simulink model "Vehicle_definitivo_validazione_2"  (R2025b)
settings: Solver=ode4  StartTime=0.0  StopTime=30  FixedStep=0.001  RelTol=1e-3
undefined symbols (not defined in the file): car, new_lotus_bump, new_lotus_roll, new_lotus_steer, posRef, rad, s, Tau_1, Tau_2, Tau_3, Tau_4, yawRef
libraries: aerolibconvert2 x28, simulink_extras x16, simulink x12, slpidlib x2, mpclib x1
(part 6 of 13)

== system Vehicle_definitivo_validazione_2/Con relaxation/Vehicle/Chassis/kinematics/FR ==
  note: mettere 2d su cmaber e toe
  Wheel_Travel : Inport
  Steer_Angle : Inport  Port=2
  Add : Sum
  Add1 : Sum  Inputs=+++
  Anti_dive : Lookup_n-D  NumberOfTableDimensions=1  BreakpointsForDimension1=[-20;-19;-18;-17;-16;-15;-14;-13;-12;-11;-10;-9;-8;-7;-6;-5;-4;-3;-2;-1;0;1;2;3;4;5;6;7;8;9;10;11;12;13;14;15;16;17;18;19;20;21;22;23;24;25;26;27;28;29;30;31;32;33;34;35;36;37;38;39;40;41;42;43;44;45;46;47;48;49;50;51;52;53;54;55;56;57;58;59;60;61;62;63;64;65;66;67;68;69;70;71;72;73;74;75]  Table=[53.85;54.03;54.22;54.4;54.59;54.77;54.96;55.15;55.34;55.53;55.72;55.92;56.11;56.31;56.5;56.7;56.9;57.1;57.3;57.5;57.71;57.91;58.12;58.32;58.53;58.74;58.95;59.16;59.38;59.59;59.81;60.03;60.24;60.46;60.69;60.91;61.13;61.36;61.59;61.81;62.04;62.28;62.51;62.74;62.98;63.22;63.46;63.7;63.94;64.18000000000001;64.43000000000001;64.68000000000001;64.92;65.17;65.43000000000001;65.68000000000001;65.94;66.19;66.45;66.72;66.98;67.23999999999999;67.51000000000001;67.78;68.05;68.31999999999999;68.59999999999999;68.87;69.15000000000001;69.43000000000001;69.72;70;70.29000000000001;70.58;70.87;71.16;71.45999999999999;71.75;72.05;72.36;72.66;72.97;73.28;73.59;73.91;74.22;74.54000000000001;74.86;75.19;75.52;75.84999999999999;76.18000000000001;76.51000000000001;76.84999999999999;77.19;77.54000000000001]/100  InternalRulePriority=Speed  RndMeth=Simplest
  Constant : Constant  Value=car.camber0_front
  Constant1 : Constant  Value=car.toe0_front
  Gain : Gain  Gain=0.222222
  IR : Lookup_n-D  NumberOfTableDimensions=1  BreakpointsForDimension1=[-20;-19;-18;-17;-16;-15;-14;-13;-12;-11;-10;-9;-8;-7;-6;-5;-4;-3;-2;-1;0;1;2;3;4;5;6;7;8;9;10;11;12;13;14;15;16;17;18;19;20;21;22;23;24;25;26;27;28;29;30;31;32;33;34;35;36;37;38;39;40;41;42;43;44;45;46;47;48;49;50;51;52;53;54;55;56;57;58;59;60;61;62;63;64;65;66;67;68;69;70;71;72;73;74;75]  Table=[0.556793;0.557414;0.558036;0.558659;0.559284;0.55991;0.5602240000000001;0.560538;0.561167;0.561167;0.561482;0.561798;0.562114;0.562114;0.562114;0.562114;0.562114;0.562114;0.562114;0.562114;0.561798;0.561798;0.561482;0.561482;0.561167;0.560852;0.560538;0.5602240000000001;0.55991;0.559284;0.558971;0.558347;0.558036;0.557414;0.557103;0.5564829999999999;0.555864;0.555247;0.554631;0.554017;0.553403;0.552792;0.552181;0.551572;0.550661;0.550055;0.549451;0.548546;0.547945;0.547046;0.546448;0.545554;0.544662;0.543774;0.543183;0.542299;0.541419;0.540541;0.539665;0.538793;0.537924;0.537057;0.536193;0.535332;0.534474;0.533618;0.532765;0.531915;0.531067;0.529942;0.529101;0.528262;0.527426;0.526593;0.525486;0.524659;0.523834;0.522739;0.521921;0.521105;0.5202909999999999;0.519211;0.5184029999999999;0.517598;0.516529;0.51573;0.514933;0.514139;0.513084;0.5122949999999999;0.511509;0.510725;0.509944;0.509165;0.508388;0.507614]  InternalRulePriority=Speed  RndMeth=Simplest
  camber : Lookup_n-D  NumberOfTableDimensions=1  BreakpointsForDimension1=[-20;-19;-18;-17;-16;-15;-14;-13;-12;-11;-10;-9;-8;-7;-6;-5;-4;-3;-2;-1;0;1;2;3;4;5;6;7;8;9;10;11;12;13;14;15;16;17;18;19;20;21;22;23;24;25;26;27;28;29;30;31;32;33;34;35;36;37;38;39;40;41;42;43;44;45;46;47;48;49;50;51;52;53;54;55;56;57;58;59;60;61;62;63;64;65;66;67;68;69;70;71;72;73;74;75]  Table=[0.17;0.13;0.08;0.04;-0.01;-0.05;-0.1;-0.15;-0.19;-0.24;-0.29;-0.33;-0.38;-0.42;-0.47;-0.52;-0.5600000000000001;-0.61;-0.66;-0.7;-0.75;-0.8;-0.84;-0.89;-0.9399999999999999;-0.98;-1.03;-1.08;-1.13;-1.17;-1.22;-1.27;-1.31;-1.36;-1.41;-1.46;-1.5;-1.55;-1.6;-1.65;-1.7;-1.74;-1.79;-1.84;-1.89;-1.94;-1.99;-2.03;-2.08;-2.13;-2.18;-2.23;-2.28;-2.33;-2.38;-2.42;-2.47;-2.52;-2.57;-2.62;-2.67;-2.72;-2.77;-2.82;-2.87;-2.92;-2.97;-3.02;-3.07;-3.12;-3.17;-3.23;-3.28;-3.33;-3.38;-3.43;-3.48;-3.53;-3.58;-3.64;-3.69;-3.74;-3.79;-3.84;-3.9;-3.95;-4;-4.05;-4.11;-4.16;-4.21;-4.27;-4.32;-4.37;-4.43;-4.48]+0.75  InternalRulePriority=Speed  RndMeth=Simplest
  steer vs toe : Lookup_n-D  NumberOfTableDimensions=1  BreakpointsForDimension1=new_lotus_steer.rack_travel  Table=new_lotus_steer.toe_angle_LHS  InternalRulePriority=Speed  RndMeth=Simplest
  toe : Lookup_n-D  NumberOfTableDimensions=1  BreakpointsForDimension1=[-20;-19;-18;-17;-16;-15;-14;-13;-12;-11;-10;-9;-8;-7;-6;-5;-4;-3;-2;-1;0;1;2;3;4;5;6;7;8;9;10;11;12;13;14;15;16;17;18;19;20;21;22;23;24;25;26;27;28;29;30;31;32;33;34;35;36;37;38;39;40;41;42;43;44;45;46;47;48;49;50;51;52;53;54;55;56;57;58;59;60;61;62;63;64;65;66;67;68;69;70;71;72;73;74;75]  Table=new_lotus_bump.front_LHS.toe  InternalRulePriority=Speed  RndMeth=Simplest
  wheelbase_change : Lookup_n-D  NumberOfTableDimensions=1  BreakpointsForDimension1=[-20;-19;-18;-17;-16;-15;-14;-13;-12;-11;-10;-9;-8;-7;-6;-5;-4;-3;-2;-1;0;1;2;3;4;5;6;7;8;9;10;11;12;13;14;15;16;17;18;19;20;21;22;23;24;25;26;27;28;29;30;31;32;33;34;35;36;37;38;39;40;41;42;43;44;45;46;47;48;49;50;51;52;53;54;55;56;57;58;59;60;61;62;63;64;65;66;67;68;69;70;71;72;73;74;75]  Table=[0.68000000000000005;0.65000000000000002;0.60999999999999999;0.56999999999999995;0.54000000000000004;0.5;0.46999999999999997;0.42999999999999999;0.40000000000000002;0.35999999999999999;0.33000000000000002;0.28999999999999998;0.26000000000000001;0.23000000000000001;0.19;0.16;0.13;0.089999999999999997;0.059999999999999998;0.029999999999999999;0;-0.029999999999999999;-0.059999999999999998;-0.089999999999999997;-0.12;-0.14999999999999999;-0.17999999999999999;-0.20999999999999999;-0.23999999999999999;-0.27000000000000002;-0.29999999999999999;-0.32000000000000001;-0.34999999999999998;-0.38;-0.40000000000000002;-0.42999999999999999;-0.46000000000000002;-0.47999999999999998;-0.51000000000000001;-0.53000000000000003;-0.56000000000000005;-0.57999999999999996;-0.60999999999999999;-0.63;-0.65000000000000002;-0.68000000000000005;-0.69999999999999996;-0.71999999999999997;-0.73999999999999999;-0.76000000000000001;-0.79000000000000004;-0.81000000000000005;-0.82999999999999996;-0.84999999999999998;-0.87;-0.89000000000000001;-0.91000000000000003;-0.92000000000000004;-0.93999999999999995;-0.95999999999999996;-0.97999999999999998;-0.98999999999999999;-1.01;-1.03;-1.04;-1.0600000000000001;-1.0700000000000001;-1.0900000000000001;-1.1000000000000001;-1.1200000000000001;-1.1299999999999999;-1.1399999999999999;-1.1499999999999999;-1.1699999999999999;-1.1799999999999999;-1.1899999999999999;-1.2;-1.21;-1.22;-1.23;-1.24;-1.25;-1.26;-1.26;-1.27;-1.28;-1.29;-1.29;-1.3;-1.3;-1.3100000000000001;-1.3100000000000001;-1.3100000000000001;-1.3200000000000001;-1.3200000000000001;-1.3200000000000001]/1000  InternalRulePriority=Speed  RndMeth=Simplest
  wb_FR : Outport
  AD_FR : Outport  Port=2
  IR_FR : Outport  Port=3
  Camber_FR : Outport  Port=4
  Toe_FR : Outport  Port=5
  wires:
  Wheel_Travel/1 -> Anti_dive/1, IR/1, toe/1, camber/1, wheelbase_change/1
  wheelbase_change/1 -> wb_FR/1
  Anti_dive/1 -> AD_FR/1
  IR/1 -> IR_FR/1
  camber/1 -> Add/2
  Constant/1 -> Add/1
  Add/1 -> Camber_FR/1
  Add1/1 -> Toe_FR/1
  Constant1/1 -> Add1/1
  toe/1 -> Add1/2
  steer vs toe/1 -> Add1/3  "toe_FR"
  Gain/1 -> steer vs toe/1
  Steer_Angle/1 -> Gain/1

== system Vehicle_definitivo_validazione_2/Con relaxation/Vehicle/Chassis/kinematics/RL ==
  Wheel_Travel : Inport
  Add : Sum
  Add2 : Sum
  Anti_squat : Lookup_n-D  NumberOfTableDimensions=1  BreakpointsForDimension1=[-20;-19;-18;-17;-16;-15;-14;-13;-12;-11;-10;-9;-8;-7;-6;-5;-4;-3;-2;-1;0;1;2;3;4;5;6;7;8;9;10;11;12;13;14;15;16;17;18;19;20;21;22;23;24;25;26;27;28;29;30;31;32;33;34;35;36;37;38;39;40;41;42;43;44;45;46;47;48;49;50;51;52;53;54;55;56;57;58;59;60;61;62;63;64;65;66;67;68;69;70;71;72;73;74;75]  Table=[53.82;53.82;53.82;53.82;53.82;53.82;53.82;53.82;53.82;53.82;53.83;53.83;53.83;53.83;53.84;53.84;53.84;53.85;53.85;53.86;53.86;53.87;53.87;53.88;53.88;53.89;53.9;53.9;53.91;53.92;53.92;53.93;53.94;53.95;53.95;53.96;53.97;53.98;53.99;54;54.01;54.01;54.02;54.03;54.04;54.05;54.06;54.07;54.08;54.09;54.1;54.11;54.12;54.13;54.15;54.16;54.17;54.18;54.19;54.2;54.21;54.22;54.23;54.24;54.25;54.27;54.28;54.29;54.3;54.31;54.32;54.33;54.34;54.35;54.36;54.37;54.38;54.39;54.4;54.41;54.42;54.43;54.44;54.45;54.46;54.47;54.48;54.49;54.49;54.5;54.51;54.52;54.52;54.53;54.54;54.54]/100  InternalRulePriority=Speed  RndMeth=Simplest
  Constant : Constant  Value=car.camber0_rear
  Constant2 : Constant  Value=car.toe0_rear
  Gain2 : Gain  Gain=-1
  IR : Lookup_n-D  NumberOfTableDimensions=1  BreakpointsForDimension1=[-20;-19;-18;-17;-16;-15;-14;-13;-12;-11;-10;-9;-8;-7;-6;-5;-4;-3;-2;-1;0;1;2;3;4;5;6;7;8;9;10;11;12;13;14;15;16;17;18;19;20;21;22;23;24;25;26;27;28;29;30;31;32;33;34;35;36;37;38;39;40;41;42;43;44;45;46;47;48;49;50;51;52;53;54;55;56;57;58;59;60;61;62;63;64;65;66;67;68;69;70;71;72;73;74;75]  Table=[0.7616000000000001;0.7616000000000001;0.7616000000000001;0.7616000000000001;0.7616000000000001;0.7616000000000001;0.7616000000000001;0.7622;0.7622;0.7628;0.7628;0.7634;0.7639;0.7645;0.7651;0.7657;0.7663;0.7669;0.7675;0.768;0.7692;0.7698;0.7704;0.7716;0.7722;0.7734;0.774;0.7746;0.7758;0.7764;0.7776;0.7782;0.7794;0.78;0.7813;0.7819;0.7831;0.7837;0.7849;0.7855;0.7868000000000001;0.7874;0.7886;0.7893;0.7905;0.7911;0.7917999999999999;0.793;0.7937;0.7943;0.7949000000000001;0.7962;0.7968;0.7974;0.7981;0.7987;0.7994;0.8;0.8;0.8006;0.8013;0.8013;0.8018999999999999;0.8018999999999999;0.8026;0.8026;0.8026;0.8026;0.8026;0.8026;0.8026;0.8018999999999999;0.8018999999999999;0.8013;0.8006;0.8;0.7994;0.7987;0.7974;0.7968;0.7955;0.7943;0.7924;0.7911;0.7893;0.7874;0.7849;0.7831;0.7806;0.7776;0.7752;0.7722;0.7685999999999999;0.7651;0.7616000000000001;0.7576000000000001]  InternalRulePriority=Speed  RndMeth=Simplest
  camber : Lookup_n-D  NumberOfTableDimensions=1  BreakpointsForDimension1=[-20;-19;-18;-17;-16;-15;-14;-13;-12;-11;-10;-9;-8;-7;-6;-5;-4;-3;-2;-1;0;1;2;3;4;5;6;7;8;9;10;11;12;13;14;15;16;17;18;19;20;21;22;23;24;25;26;27;28;29;30;31;32;33;34;35;36;37;38;39;40;41;42;43;44;45;46;47;48;49;50;51;52;53;54;55;56;57;58;59;60;61;62;63;64;65;66;67;68;69;70;71;72;73;74;75]  Table=[0.79000000000000004;0.75;0.70999999999999996;0.67000000000000004;0.63;0.58999999999999997;0.55000000000000004;0.51000000000000001;0.46999999999999997;0.42999999999999999;0.39000000000000001;0.34999999999999998;0.31;0.27000000000000002;0.23999999999999999;0.20000000000000001;0.16;0.12;0.080000000000000002;0.040000000000000001;0;-0.040000000000000001;-0.080000000000000002;-0.12;-0.16;-0.20000000000000001;-0.23999999999999999;-0.27000000000000002;-0.31;-0.34999999999999998;-0.39000000000000001;-0.42999999999999999;-0.46999999999999997;-0.51000000000000001;-0.55000000000000004;-0.58999999999999997;-0.63;-0.67000000000000004;-0.70999999999999996;-0.75;-0.79000000000000004;-0.82999999999999996;-0.85999999999999999;-0.90000000000000002;-0.93999999999999995;-0.97999999999999998;-1.02;-1.0600000000000001;-1.1000000000000001;-1.1399999999999999;-1.1799999999999999;-1.22;-1.26;-1.3;-1.3400000000000001;-1.3799999999999999;-1.4199999999999999;-1.46;-1.5;-1.54;-1.5800000000000001;-1.6200000000000001;-1.6599999999999999;-1.7;-1.74;-1.78;-1.8200000000000001;-1.8600000000000001;-1.8999999999999999;-1.9399999999999999;-1.98;-2.02;-2.0699999999999998;-2.1099999999999999;-2.1499999999999999;-2.1899999999999999;-2.23;-2.27;-2.3100000000000001;-2.3500000000000001;-2.3900000000000001;-2.4399999999999999;-2.48;-2.52;-2.5600000000000001;-2.6000000000000001;-2.6400000000000001;-2.6899999999999999;-2.73;-2.77;-2.8100000000000001;-2.8500000000000001;-2.8999999999999999;-2.9399999999999999;-2.98;-3.02]  InternalRulePriority=Speed  RndMeth=Simplest
  toe : Lookup_n-D  NumberOfTableDimensions=1  BreakpointsForDimension1=new_lotus_bump.wheeltravel  Table=new_lotus_bump.rear_LHS.toe  InternalRulePriority=Speed  RndMeth=Simplest
  wheelbase_change : Lookup_n-D  NumberOfTableDimensions=1  BreakpointsForDimension1=[-20;-19;-18;-17;-16;-15;-14;-13;-12;-11;-10;-9;-8;-7;-6;-5;-4;-3;-2;-1;0;1;2;3;4;5;6;7;8;9;10;11;12;13;14;15;16;17;18;19;20;21;22;23;24;25;26;27;28;29;30;31;32;33;34;35;36;37;38;39;40;41;42;43;44;45;46;47;48;49;50;51;52;53;54;55;56;57;58;59;60;61;62;63;64;65;66;67;68;69;70;71;72;73;74;75]  Table=[-2.1899999999999999;-2.0800000000000001;-1.97;-1.8600000000000001;-1.74;-1.6299999999999999;-1.52;-1.4099999999999999;-1.3;-1.1899999999999999;-1.0800000000000001;-0.96999999999999997;-0.85999999999999999;-0.75;-0.65000000000000002;-0.54000000000000004;-0.42999999999999999;-0.32000000000000001;-0.20999999999999999;-0.11;0;0.11;0.20999999999999999;0.32000000000000001;0.41999999999999998;0.53000000000000003;0.63;0.73999999999999999;0.83999999999999997;0.94999999999999996;1.05;1.1599999999999999;1.26;1.3600000000000001;1.47;1.5700000000000001;1.6699999999999999;1.77;1.8700000000000001;1.98;2.0800000000000001;2.1800000000000002;2.2799999999999998;2.3799999999999999;2.48;2.5800000000000001;2.6800000000000002;2.7799999999999998;2.8799999999999999;2.9700000000000002;3.0699999999999998;3.1699999999999999;3.27;3.3700000000000001;3.46;3.5600000000000001;3.6600000000000001;3.7599999999999998;3.8500000000000001;3.9500000000000002;4.04;4.1399999999999997;4.2400000000000002;4.3300000000000001;4.4299999999999997;4.5199999999999996;4.6100000000000003;4.71;4.7999999999999998;4.9000000000000004;4.9900000000000002;5.0800000000000001;5.1799999999999997;5.2699999999999996;5.3600000000000003;5.4500000000000002;5.5499999999999998;5.6399999999999997;5.7300000000000004;5.8200000000000003;5.9100000000000001;6;6.0899999999999999;6.1799999999999997;6.2699999999999996;6.3600000000000003;6.4500000000000002;6.54;6.6299999999999999;6.7199999999999998;6.8099999999999996;6.9000000000000004;6.9900000000000002;7.0700000000000003;7.1600000000000001;7.25]/1000  InternalRulePriority=Speed  RndMeth=Simplest
  wb_RL : Outport
  AS_RL : Outport  Port=2
  IR_RL : Outport  Port=3
  Camber_RL : Outport  Port=4
  Toe_RL : Outport  Port=5
  wires:
  Wheel_Travel/1 -> Anti_squat/1, wheelbase_change/1, IR/1, toe/1, camber/1
  wheelbase_change/1 -> wb_RL/1
  Anti_squat/1 -> AS_RL/1
  IR/1 -> IR_RL/1
  Add/1 -> Camber_RL/1
  Constant/1 -> Add/1
  camber/1 -> Add/2
  Constant2/1 -> Add2/1
  Add2/1 -> Toe_RL/1
  toe/1 -> Gain2/1
  Gain2/1 -> Add2/2

== system Vehicle_definitivo_validazione_2/Con relaxation/Vehicle/Chassis/kinematics/RR ==
  Wheel_Travel : Inport
  Add : Sum
  Add2 : Sum
  Anti_squat : Lookup_n-D  NumberOfTableDimensions=1  BreakpointsForDimension1=[-20;-19;-18;-17;-16;-15;-14;-13;-12;-11;-10;-9;-8;-7;-6;-5;-4;-3;-2;-1;0;1;2;3;4;5;6;7;8;9;10;11;12;13;14;15;16;17;18;19;20;21;22;23;24;25;26;27;28;29;30;31;32;33;34;35;36;37;38;39;40;41;42;43;44;45;46;47;48;49;50;51;52;53;54;55;56;57;58;59;60;61;62;63;64;65;66;67;68;69;70;71;72;73;74;75]  Table=[53.82;53.82;53.82;53.82;53.82;53.82;53.82;53.82;53.82;53.82;53.83;53.83;53.83;53.83;53.84;53.84;53.84;53.85;53.85;53.86;53.86;53.87;53.87;53.88;53.88;53.89;53.9;53.9;53.91;53.92;53.92;53.93;53.94;53.95;53.95;53.96;53.97;53.98;53.99;54;54.01;54.01;54.02;54.03;54.04;54.05;54.06;54.07;54.08;54.09;54.1;54.11;54.12;54.13;54.15;54.16;54.17;54.18;54.19;54.2;54.21;54.22;54.23;54.24;54.25;54.27;54.28;54.29;54.3;54.31;54.32;54.33;54.34;54.35;54.36;54.37;54.38;54.39;54.4;54.41;54.42;54.43;54.44;54.45;54.46;54.47;54.48;54.49;54.49;54.5;54.51;54.52;54.52;54.53;54.54;54.54]/100  InternalRulePriority=Speed  RndMeth=Simplest
  Constant : Constant  Value=car.camber0_rear
  Constant2 : Constant  Value=car.toe0_rear
  IR : Lookup_n-D  NumberOfTableDimensions=1  BreakpointsForDimension1=[-20;-19;-18;-17;-16;-15;-14;-13;-12;-11;-10;-9;-8;-7;-6;-5;-4;-3;-2;-1;0;1;2;3;4;5;6;7;8;9;10;11;12;13;14;15;16;17;18;19;20;21;22;23;24;25;26;27;28;29;30;31;32;33;34;35;36;37;38;39;40;41;42;43;44;45;46;47;48;49;50;51;52;53;54;55;56;57;58;59;60;61;62;63;64;65;66;67;68;69;70;71;72;73;74;75]  Table=[0.7616000000000001;0.7616000000000001;0.7616000000000001;0.7616000000000001;0.7616000000000001;0.7616000000000001;0.7616000000000001;0.7622;0.7622;0.7628;0.7628;0.7634;0.7639;0.7645;0.7651;0.7657;0.7663;0.7669;0.7675;0.768;0.7692;0.7698;0.7704;0.7716;0.7722;0.7734;0.774;0.7746;0.7758;0.7764;0.7776;0.7782;0.7794;0.78;0.7813;0.7819;0.7831;0.7837;0.7849;0.7855;0.7868000000000001;0.7874;0.7886;0.7893;0.7905;0.7911;0.7917999999999999;0.793;0.7937;0.7943;0.7949000000000001;0.7962;0.7968;0.7974;0.7981;0.7987;0.7994;0.8;0.8;0.8006;0.8013;0.8013;0.8018999999999999;0.8018999999999999;0.8026;0.8026;0.8026;0.8026;0.8026;0.8026;0.8026;0.8018999999999999;0.8018999999999999;0.8013;0.8006;0.8;0.7994;0.7987;0.7974;0.7968;0.7955;0.7943;0.7924;0.7911;0.7893;0.7874;0.7849;0.7831;0.7806;0.7776;0.7752;0.7722;0.7685999999999999;0.7651;0.7616000000000001;0.7576000000000001]  InternalRulePriority=Speed  RndMeth=Simplest
  camber : Lookup_n-D  NumberOfTableDimensions=1  BreakpointsForDimension1=[-20;-19;-18;-17;-16;-15;-14;-13;-12;-11;-10;-9;-8;-7;-6;-5;-4;-3;-2;-1;0;1;2;3;4;5;6;7;8;9;10;11;12;13;14;15;16;17;18;19;20;21;22;23;24;25;26;27;28;29;30;31;32;33;34;35;36;37;38;39;40;41;42;43;44;45;46;47;48;49;50;51;52;53;54;55;56;57;58;59;60;61;62;63;64;65;66;67;68;69;70;71;72;73;74;75]  Table=[0.79000000000000004;0.75;0.70999999999999996;0.67000000000000004;0.63;0.58999999999999997;0.55000000000000004;0.51000000000000001;0.46999999999999997;0.42999999999999999;0.39000000000000001;0.34999999999999998;0.31;0.27000000000000002;0.23999999999999999;0.20000000000000001;0.16;0.12;0.080000000000000002;0.040000000000000001;0;-0.040000000000000001;-0.080000000000000002;-0.12;-0.16;-0.20000000000000001;-0.23999999999999999;-0.27000000000000002;-0.31;-0.34999999999999998;-0.39000000000000001;-0.42999999999999999;-0.46999999999999997;-0.51000000000000001;-0.55000000000000004;-0.58999999999999997;-0.63;-0.67000000000000004;-0.70999999999999996;-0.75;-0.79000000000000004;-0.82999999999999996;-0.85999999999999999;-0.90000000000000002;-0.93999999999999995;-0.97999999999999998;-1.02;-1.0600000000000001;-1.1000000000000001;-1.1399999999999999;-1.1799999999999999;-1.22;-1.26;-1.3;-1.3400000000000001;-1.3799999999999999;-1.4199999999999999;-1.46;-1.5;-1.54;-1.5800000000000001;-1.6200000000000001;-1.6599999999999999;-1.7;-1.74;-1.78;-1.8200000000000001;-1.8600000000000001;-1.8999999999999999;-1.9399999999999999;-1.98;-2.02;-2.0699999999999998;-2.1099999999999999;-2.1499999999999999;-2.1899999999999999;-2.23;-2.27;-2.3100000000000001;-2.3500000000000001;-2.3900000000000001;-2.4399999999999999;-2.48;-2.52;-2.5600000000000001;-2.6000000000000001;-2.6400000000000001;-2.6899999999999999;-2.73;-2.77;-2.8100000000000001;-2.8500000000000001;-2.8999999999999999;-2.9399999999999999;-2.98;-3.02]  InternalRulePriority=Speed  RndMeth=Simplest
  toe : Lookup_n-D  NumberOfTableDimensions=1  BreakpointsForDimension1=new_lotus_bump.wheeltravel  Table=new_lotus_bump.rear_LHS.toe  InternalRulePriority=Speed  RndMeth=Simplest
  wheelbase_change : Lookup_n-D  NumberOfTableDimensions=1  BreakpointsForDimension1=[-20;-19;-18;-17;-16;-15;-14;-13;-12;-11;-10;-9;-8;-7;-6;-5;-4;-3;-2;-1;0;1;2;3;4;5;6;7;8;9;10;11;12;13;14;15;16;17;18;19;20;21;22;23;24;25;26;27;28;29;30;31;32;33;34;35;36;37;38;39;40;41;42;43;44;45;46;47;48;49;50;51;52;53;54;55;56;57;58;59;60;61;62;63;64;65;66;67;68;69;70;71;72;73;74;75]  Table=[-2.1899999999999999;-2.0800000000000001;-1.97;-1.8600000000000001;-1.74;-1.6299999999999999;-1.52;-1.4099999999999999;-1.3;-1.1899999999999999;-1.0800000000000001;-0.96999999999999997;-0.85999999999999999;-0.75;-0.65000000000000002;-0.54000000000000004;-0.42999999999999999;-0.32000000000000001;-0.20999999999999999;-0.11;0;0.11;0.20999999999999999;0.32000000000000001;0.41999999999999998;0.53000000000000003;0.63;0.73999999999999999;0.83999999999999997;0.94999999999999996;1.05;1.1599999999999999;1.26;1.3600000000000001;1.47;1.5700000000000001;1.6699999999999999;1.77;1.8700000000000001;1.98;2.0800000000000001;2.1800000000000002;2.2799999999999998;2.3799999999999999;2.48;2.5800000000000001;2.6800000000000002;2.7799999999999998;2.8799999999999999;2.9700000000000002;3.0699999999999998;3.1699999999999999;3.27;3.3700000000000001;3.46;3.5600000000000001;3.6600000000000001;3.7599999999999998;3.8500000000000001;3.9500000000000002;4.04;4.1399999999999997;4.2400000000000002;4.3300000000000001;4.4299999999999997;4.5199999999999996;4.6100000000000003;4.71;4.7999999999999998;4.9000000000000004;4.9900000000000002;5.0800000000000001;5.1799999999999997;5.2699999999999996;5.3600000000000003;5.4500000000000002;5.5499999999999998;5.6399999999999997;5.7300000000000004;5.8200000000000003;5.9100000000000001;6;6.0899999999999999;6.1799999999999997;6.2699999999999996;6.3600000000000003;6.4500000000000002;6.54;6.6299999999999999;6.7199999999999998;6.8099999999999996;6.9000000000000004;6.9900000000000002;7.0700000000000003;7.1600000000000001;7.25]/1000  InternalRulePriority=Speed  RndMeth=Simplest
  wb_RR : Outport
  AS_RR : Outport  Port=2
  IR_RR : Outport  Port=3
  Camber_RR : Outport  Port=4
  Toe_RR : Outport  Port=5
  wires:
  Wheel_Travel/1 -> Anti_squat/1, wheelbase_change/1, IR/1, camber/1, toe/1
  wheelbase_change/1 -> wb_RR/1
  Anti_squat/1 -> AS_RR/1
  IR/1 -> IR_RR/1
  Add/1 -> Camber_RR/1
  Constant/1 -> Add/1
  camber/1 -> Add/2
  Constant2/1 -> Add2/1
  Add2/1 -> Toe_RR/1
  toe/1 -> Add2/2

== system Vehicle_definitivo_validazione_2/Con relaxation/Vehicle/Chassis/kinematics/Subsystem ==
  Heave_F : Inport
  Roll_F : Inport  Port=2
  Add : Sum
  Constant : Constant  Value=car.tf
  Constant1 : Constant  Value=car.tf
  Divide : Product  Inputs=*/
  Gain : Gain  Gain=-1
  H_rc : Lookup_n-D  BreakpointsForDimension1=[1:3]  BreakpointsForDimension2=[1:3]  InternalRulePriority=Speed  RndMeth=Simplest
      settings: InputPortMap=u0,u1
  Radians to Degrees : simulink_extras/Transformations/Radians to Degrees
  Tan : Trigonometry  Operator=atan
  track_change : Lookup_n-D  NumberOfTableDimensions=1  BreakpointsForDimension1=new_lotus_roll.roll_angle  Table=new_lotus_roll.front_LHS.half_track_change/1000  InternalRulePriority=Speed  RndMeth=Simplest
  h_rc_f : Outport
  tf : Outport  Port=2
  wires:
  Heave_F/1 -> H_rc/1
  track_change/1 -> Add/1  "track_change"
  Constant/1 -> Add/2
  Add/1 -> tf/1  "tf"
  H_rc/1 -> h_rc_f/1  "h_rc_f"
  Roll_F/1 -> Divide/1
  Divide/1 -> Tan/1
  Tan/1 -> Radians to Degrees/1
  Gain/1 -> track_change/1, H_rc/2
  Constant1/1 -> Divide/2
  Radians to Degrees/1 -> Gain/1

== system Vehicle_definitivo_validazione_2/Con relaxation/Vehicle/Chassis/kinematics/Subsystem1 ==
  Heave_R : Inport
  Roll_R : Inport  Port=2
  Add : Sum
  Constant : Constant  Value=car.tr
  Constant1 : Constant  Value=car.tr
  Divide : Product  Inputs=*/
  Gain : Gain  Gain=-1
  H_rc : Lookup_n-D  BreakpointsForDimension1=[1:3]  BreakpointsForDimension2=[1:3]  InternalRulePriority=Speed  RndMeth=Simplest
      settings: InputPortMap=u0,u1
  Radians to Degrees : simulink_extras/Transformations/Radians to Degrees
  Tan : Trigonometry  Operator=atan
  track_change : Lookup_n-D  NumberOfTableDimensions=1  BreakpointsForDimension1=new_lotus_roll.roll_angle  Table=new_lotus_roll.rear_LHS.half_track_change/1000  InternalRulePriority=Speed  RndMeth=Simplest
  h_rc_r : Outport
  tr : Outport  Port=2
  wires:
  track_change/1 -> Add/1  "track_change"
  Constant/1 -> Add/2
  H_rc/1 -> h_rc_r/1  "h_rc_r"
  Roll_R/1 -> Divide/1
  Heave_R/1 -> H_rc/1
  Divide/1 -> Tan/1
  Add/1 -> tr/1  "tr"
  Gain/1 -> track_change/1, H_rc/2
  Constant1/1 -> Divide/2
  Tan/1 -> Radians to Degrees/1
  Radians to Degrees/1 -> Gain/1

== system Vehicle_definitivo_validazione_2/Con relaxation/Vehicle/Powertrain/pwt con clutch/Engine ==
  w_ICE : Inport
  tps : Inport  Port=2
  1-D Lookup Table : Lookup_n-D  NumberOfTableDimensions=1  BreakpointsForDimension1=[0 car.limitatore car.limitatore+300]  Table=[1 1 0]  InternalRulePriority=Speed  RndMeth=Simplest
  2-D Lookup Table : Lookup_n-D  BreakpointsForDimension1=[0;4000;4500;5000;5500;6000;6500;7000;7500;8000;8500;9000;9500;10000;10500;11000;11500;12000]  BreakpointsForDimension2=[0;0.20000000000000001;0.25;0.29999999999999999;0.34999999999999998;0.40000000000000002;0.45000000000000001;0.5;0.59999999999999998;0.69999999999999996;0.80000000000000004;1]  Table=car.engine.lut  InternalRulePriority=Speed  RndMeth=Simplest
      settings: InputPortMap=u0,u1
  Limiter : Saturate  UpperLimit=12500  LowerLimit=4000
  Product : Product
  T_ICE : Outport
  wires:
  tps/1 -> 2-D Lookup Table/2
  Limiter/1 -> 2-D Lookup Table/1
  w_ICE/1 -> Limiter/1, 1-D Lookup Table/1
  1-D Lookup Table/1 -> Product/1
  2-D Lookup Table/1 -> Product/2
  Product/1 -> T_ICE/1

== system Vehicle_definitivo_validazione_2/Con relaxation/Vehicle/Powertrain/pwt con clutch/Transmission ==
  T_ICE : Inport
  gear : Inport  Port=2
  1-D Lookup Table2 : Lookup_n-D  NumberOfTableDimensions=1  BreakpointsForDimension1=[1;2;3;4]  Table=[Tau_1; Tau_2; Tau_3; Tau_4]  InternalRulePriority=Speed  RndMeth=Simplest
  Gain1 : Gain  Gain=car.eta_pwt
  Product1 : Product
  T_rear : Outport
  wires:
  Gain1/1 -> T_rear/1
  Product1/1 -> Gain1/1
  T_ICE/1 -> Product1/2
  1-D Lookup Table2/1 -> Product1/1
  gear/1 -> 1-D Lookup Table2/1

== system Vehicle_definitivo_validazione_2/Con relaxation/Vehicle/Powertrain/pwt senza clutch/Engine ==
  w_ICE : Inport
  tps : Inport  Port=2
  1-D Lookup Table : Lookup_n-D  NumberOfTableDimensions=1  BreakpointsForDimension1=[0 car.limitatore car.limitatore+300]  Table=[1 1 0]  InternalRulePriority=Speed  RndMeth=Simplest
  2-D Lookup Table : Lookup_n-D  BreakpointsForDimension1=[0;4000;4500;5000;5500;6000;6500;7000;7500;8000;8500;9000;9500;10000;10500;11000;11500;12000]  BreakpointsForDimension2=[0;0.20000000000000001;0.25;0.29999999999999999;0.34999999999999998;0.40000000000000002;0.45000000000000001;0.5;0.59999999999999998;0.69999999999999996;0.80000000000000004;1]  Table=car.engine.lut  InternalRulePriority=Speed  RndMeth=Simplest
      settings: InputPortMap=u0,u1
  Limiter : Saturate  UpperLimit=12500  LowerLimit=4000
  Product : Product
  T_ICE : Outport
  wires:
  tps/1 -> 2-D Lookup Table/2
  Limiter/1 -> 2-D Lookup Table/1
  w_ICE/1 -> Limiter/1, 1-D Lookup Table/1
  1-D Lookup Table/1 -> Product/1
  2-D Lookup Table/1 -> Product/2
  Product/1 -> T_ICE/1

== system Vehicle_definitivo_validazione_2/Con relaxation/Vehicle/Powertrain/pwt senza clutch/Transmission ==
  T_ICE : Inport
  gear : Inport  Port=2
  1-D Lookup Table2 : Lookup_n-D  NumberOfTableDimensions=1  BreakpointsForDimension1=[1;2;3;4]  Table=[Tau_1; Tau_2; Tau_3; Tau_4]  InternalRulePriority=Speed  RndMeth=Simplest
  Gain1 : Gain  Gain=car.eta_pwt
  Product1 : Product
  T_rear : Outport
  wires:
  Gain1/1 -> T_rear/1
  Product1/1 -> Gain1/1
  T_ICE/1 -> Product1/2
  1-D Lookup Table2/1 -> Product1/1
  gear/1 -> 1-D Lookup Table2/1

== system Vehicle_definitivo_validazione_2/Driver in the Loop/Vehicle/Chassis/Damper/FL ==
  V_FL : Inport
  Add : Sum
  Add1 : Sum
  Add2 : Sum
  Front compression min : Lookup_n-D  NumberOfTableDimensions=1  BreakpointsForDimension1=|  Table=|  InternalRulePriority=Speed  RndMeth=Simplest
      BreakpointsForDimension1=|
      | [0;0.025;0.051;0.076;0.102;0.127;0.152;0.178;0.203;0.229;0.254;0.279;0.305
      | ]
      Table=|
      | [0; 240.204;
      | 231.307;
      | 226.859;
      | 226.859;
      | 231.307;
      | 231.307;
      | 235.756;
      | 240.204;
      | 240.204;
      | 244.652;
      | 249.100;
      | 253.549]
  Gain : Gain  Gain=-1
  Gain1 : Gain  Gain=-1
  Gain2 : Gain  Gain=car.click_comp_F/car.click_tot_comp_F
  Gain3 : Gain  Gain=car.click_reb_F/car.click_tot_reb_F
  Saturation : Saturate  UpperLimit=inf  LowerLimit=0
  Saturation1 : Saturate  UpperLimit=0  LowerLimit=-inf
  Subtract : Sum  Inputs=+-
  Subtract1 : Sum  Inputs=+-
  front compression max : Lookup_n-D  NumberOfTableDimensions=1  BreakpointsForDimension1=|  Table=|  InternalRulePriority=Speed  RndMeth=Simplest
      BreakpointsForDimension1=|
      | [0;0.025;0.051;0.076;0.102;0.127;0.152;0.178;0.203;0.229;0.254;0.279;0.305
      | ]
      Table=|
      | [0;782.887;
      | 898.540;
      | 956.367;
      | 978.608;
      | 1000.850;
      | 1018.642;
      | 1058.676;
      | 1085.366;
      | 1107.607;
      | 1147.641
      | ;1178.778;1214.364
      | ]
  front rebound max : Lookup_n-D  NumberOfTableDimensions=1  BreakpointsForDimension1=|  Table=|  InternalRulePriority=Speed  RndMeth=Simplest
      BreakpointsForDimension1=|
      | [0;0.025;0.051;0.076;0.102;0.127;0.152;0.178;0.203;0.229;0.254;0.279;0.305
      | ]
      Table=|
      | [0; 266.893;
      | 333.617;
      | 360.306;
      | 373.650;
      | 391.443;
      | 409.236;
      | 422.581;
      | 444.822;
      | 467.063;
      | 480.408;
      | 493.752;
      | 511.545]
  front rebound min : Lookup_n-D  NumberOfTableDimensions=1  BreakpointsForDimension1=|  Table=|  InternalRulePriority=Speed  RndMeth=Simplest
      BreakpointsForDimension1=|
      | [0;0.025;0.051;0.076;0.102;0.127;0.152;0.178;0.203;0.229;0.254;0.279;0.305
      | ]
      Table=|
      | [0; 40.034;
      | 26.689;
      | 17.793;
      | 8.896;
      | 4.448;
      | 4.448;
      | 4.448;
      | 8.896;
      | 35.586;
      | 31.138;
      | 53.379;
      | 26.689]
  F_FL : Outport
  wires:
  Front compression min/1 -> Subtract/2, Add1/2
  front rebound min/1 -> Add2/2, Subtract1/2
  Subtract1/1 -> Gain3/1
  Gain3/1 -> Add2/1
  Subtract/1 -> Gain2/1
  Gain2/1 -> Add1/1
  front compression max/1 -> Subtract/1
  front rebound max/1 -> Subtract1/1
  Saturation/1 -> front compression max/1, Front compression min/1
  Gain1/1 -> front rebound min/1, front rebound max/1
  Add2/1 -> Gain/1
  V_FL/1 -> Saturation/1, Saturation1/1
  Saturation1/1 -> Gain1/1
  Gain/1 -> Add/2
  Add1/1 -> Add/1
  Add/1 -> F_FL/1

== system Vehicle_definitivo_validazione_2/Driver in the Loop/Vehicle/Chassis/Damper/FR ==
  V_FR : Inport
  Add : Sum
  Add1 : Sum
  Add2 : Sum
  Front compression min : Lookup_n-D  NumberOfTableDimensions=1  BreakpointsForDimension1=|  Table=|  InternalRulePriority=Speed  RndMeth=Simplest
      BreakpointsForDimension1=|
      | [0;0.025;0.051;0.076;0.102;0.127;0.152;0.178;0.203;0.229;0.254;0.279;0.305
      | ]
      Table=|
      | [0; 240.204;
      | 231.307;
      | 226.859;
      | 226.859;
      | 231.307;
      | 231.307;
      | 235.756;
      | 240.204;
      | 240.204;
      | 244.652;
      | 249.100;
      | 253.549]
  Gain : Gain  Gain=-1
  Gain1 : Gain  Gain=-1
  Gain2 : Gain  Gain=car.click_comp_F/car.click_tot_comp_F
  Gain3 : Gain  Gain=car.click_reb_F/car.click_tot_reb_F
  Saturation : Saturate  UpperLimit=inf  LowerLimit=0
  Saturation1 : Saturate  UpperLimit=0  LowerLimit=-inf
  Subtract : Sum  Inputs=+-
  Subtract1 : Sum  Inputs=+-
  front compression max : Lookup_n-D  NumberOfTableDimensions=1  BreakpointsForDimension1=|  Table=|  InternalRulePriority=Speed  RndMeth=Simplest
      BreakpointsForDimension1=|
      | [0;0.025;0.051;0.076;0.102;0.127;0.152;0.178;0.203;0.229;0.254;0.279;0.305
      | ]
      Table=|
      | [0;782.887;
      | 898.540;
      | 956.367;
      | 978.608;
      | 1000.850;
      | 1018.642;
      | 1058.676;
      | 1085.366;
      | 1107.607;
      | 1147.641
      | ;1178.778;1214.364
      | ]
  front rebound max : Lookup_n-D  NumberOfTableDimensions=1  BreakpointsForDimension1=|  Table=|  InternalRulePriority=Speed  RndMeth=Simplest
      BreakpointsForDimension1=|
      | [0;0.025;0.051;0.076;0.102;0.127;0.152;0.178;0.203;0.229;0.254;0.279;0.305
      | ]
      Table=|
      | [0; 266.893;
      | 333.617;
      | 360.306;
      | 373.650;
      | 391.443;
      | 409.236;
      | 422.581;
      | 444.822;
      | 467.063;
      | 480.408;
      | 493.752;
      | 511.545]
  front rebound min : Lookup_n-D  NumberOfTableDimensions=1  BreakpointsForDimension1=|  Table=|  InternalRulePriority=Speed  RndMeth=Simplest
      BreakpointsForDimension1=|
      | [0;0.025;0.051;0.076;0.102;0.127;0.152;0.178;0.203;0.229;0.254;0.279;0.305
      | ]
      Table=|
      | [0; 40.034;
      | 26.689;
      | 17.793;
      | 8.896;
      | 4.448;
      | 4.448;
      | 4.448;
      | 8.896;
      | 35.586;
      | 31.138;
      | 53.379;
      | 26.689]
  F_FR : Outport
  wires:
  Front compression min/1 -> Subtract/2, Add1/2
  front rebound min/1 -> Add2/2, Subtract1/2
  Subtract1/1 -> Gain3/1
  Gain3/1 -> Add2/1
  Subtract/1 -> Gain2/1
  Gain2/1 -> Add1/1
  front compression max/1 -> Subtract/1
  front rebound max/1 -> Subtract1/1
  Saturation/1 -> front compression max/1, Front compression min/1
  Gain1/1 -> front rebound min/1, front rebound max/1
  Add2/1 -> Gain/1
  V_FR/1 -> Saturation/1, Saturation1/1
  Saturation1/1 -> Gain1/1
  Gain/1 -> Add/2
  Add1/1 -> Add/1
  Add/1 -> F_FR/1

== system Vehicle_definitivo_validazione_2/Driver in the Loop/Vehicle/Chassis/Damper/RL ==
  V_RL : Inport
  Add : Sum
  Add1 : Sum
  Add2 : Sum
  Gain : Gain  Gain=-1
  Gain1 : Gain  Gain=-1
  Gain2 : Gain  Gain=car.click_comp_R/car.click_tot_comp_R
  Gain3 : Gain  Gain=car.click_reb_R/car.click_tot_reb_R
  Rear Compression max : Lookup_n-D  NumberOfTableDimensions=1  BreakpointsForDimension1=|  Table=|  InternalRulePriority=Speed  RndMeth=Simplest
      BreakpointsForDimension1=|
      | [0; 0.025;
      | 0.051;
      | 0.076;
      | 0.102;
      | 0.127;
      | 0.152;
      | 0.178;
      | 0.203;
      | 0.229;
      | 0.254;
      | 0.279;
      | 0.305
      | ]
      Table=|
      | [0; 667.233;
      | 782.887;
      | 885.196;
      | 934.126;
      | 965.264;
      | 996.401;
      | 1018.642;
      | 1049.780;
      | 1076.469;
      | 1112.055;
      | 1138.744;  1169.882
      | ]
  Rear Compression min : Lookup_n-D  NumberOfTableDimensions=1  BreakpointsForDimension1=|  Table=|  InternalRulePriority=Speed  RndMeth=Simplest
      BreakpointsForDimension1=|
      | [0; 0.025;
      | 0.051;
      | 0.076;
      | 0.102;
      | 0.127;
      | 0.152;
      | 0.178;
      | 0.203;
      | 0.229;
      | 0.254;
      | 0.279;
      | 0.305
      | ]
      Table=|
      | [0; 213.515;
      | 204.618;
      | 200.170;
      | 195.722;
      | 195.722;
      | 200.170;
      | 200.170;
      | 204.618;
      | 204.618;
      | 209.066;
      | 213.515;
      | 213.515
      | ]
  Rear Rebound max : Lookup_n-D  NumberOfTableDimensions=1  BreakpointsForDimension1=|  Table=|  InternalRulePriority=Speed  RndMeth=Simplest
      BreakpointsForDimension1=|
      | [0; 0.025;
      | 0.051;
      | 0.076;
      | 0.102;
      | 0.127;
      | 0.152;
      | 0.178;
      | 0.203;
      | 0.229;
      | 0.254;
      | 0.279;
      | 0.305
      | ]
      Table=|
      | [0; 124.550;
      | 191.273;
      | 244.652;
      | 284.686;
      | 329.168;
      | 369.202;
      | 391.443;
      | 413.684;
      | 431.477;
      | 449.270;
      | 458.167;
      | 471.511
      | ]
  Rear Rebound min : Lookup_n-D  NumberOfTableDimensions=1  BreakpointsForDimension1=|  Table=|  InternalRulePriority=Speed  RndMeth=Simplest
      BreakpointsForDimension1=|
      | [0; 0.025;
      | 0.051;
      | 0.076;
      | 0.102;
      | 0.127;
      | 0.152;
      | 0.178;
      | 0.203;
      | 0.229;
      | 0.254;
      | 0.279;
      | 0.305
      | ]
      Table=|
      | [0; 35.586;
      | 48.930;
      | 53.379;
      | 53.379;
      | 48.930;
      | 48.930;
      | 48.930;
      | 48.930;
      | 48.930;
      | 48.930;
      | 48.930;
      | 48.930
      | ]
  Saturation : Saturate  UpperLimit=inf  LowerLimit=0
  Saturation1 : Saturate  UpperLimit=0  LowerLimit=-inf
  Subtract : Sum  Inputs=+-
  Subtract1 : Sum  Inputs=+-
  F_RL : Outport
  wires:
  Rear Compression min/1 -> Subtract/2, Add1/2
  Rear Rebound min/1 -> Add2/2, Subtract1/2
  Subtract1/1 -> Gain3/1
  Gain3/1 -> Add2/1
  Subtract/1 -> Gain2/1
  Gain2/1 -> Add1/1
  Rear Compression max/1 -> Subtract/1
  Rear Rebound max/1 -> Subtract1/1
  Saturation/1 -> Rear Compression min/1, Rear Compression max/1
  Gain1/1 -> Rear Rebound min/1, Rear Rebound max/1
  Add2/1 -> Gain/1
  V_RL/1 -> Saturation/1, Saturation1/1
  Saturation1/1 -> Gain1/1
  Gain/1 -> Add/2
  Add1/1 -> Add/1
  Add/1 -> F_RL/1

== system Vehicle_definitivo_validazione_2/Driver in the Loop/Vehicle/Chassis/Damper/RR ==
  V_RR : Inport
  Add : Sum
  Add1 : Sum
  Add2 : Sum
  Gain : Gain  Gain=-1
  Gain1 : Gain  Gain=-1
  Gain2 : Gain  Gain=car.click_comp_R/car.click_tot_comp_R
  Gain3 : Gain  Gain=car.click_reb_R/car.click_tot_reb_R
  Rear Compression max : Lookup_n-D  NumberOfTableDimensions=1  BreakpointsForDimension1=|  Table=|  InternalRulePriority=Speed  RndMeth=Simplest
      BreakpointsForDimension1=|
      | [0; 0.025;
      | 0.051;
      | 0.076;
      | 0.102;
      | 0.127;
      | 0.152;
      | 0.178;
      | 0.203;
      | 0.229;
      | 0.254;
      | 0.279;
      | 0.305
      | ]
      Table=|
      | [0; 667.233;
      | 782.887;
      | 885.196;
      | 934.126;
      | 965.264;
      | 996.401;
      | 1018.642;
      | 1049.780;
      | 1076.469;
      | 1112.055;
      | 1138.744;  1169.882
      | ]
  Rear Compression min : Lookup_n-D  NumberOfTableDimensions=1  BreakpointsForDimension1=|  Table=|  InternalRulePriority=Speed  RndMeth=Simplest
      BreakpointsForDimension1=|
      | [0; 0.025;
      | 0.051;
      | 0.076;
      | 0.102;
      | 0.127;
      | 0.152;
      | 0.178;
      | 0.203;
      | 0.229;
      | 0.254;
      | 0.279;
      | 0.305
      | ]
      Table=|
      | [0; 213.515;
      | 204.618;
      | 200.170;
      | 195.722;
      | 195.722;
      | 200.170;
      | 200.170;
      | 204.618;
      | 204.618;
      | 209.066;
      | 213.515;
      | 213.515
      | ]
  Rear Rebound max : Lookup_n-D  NumberOfTableDimensions=1  BreakpointsForDimension1=|  Table=|  InternalRulePriority=Speed  RndMeth=Simplest
      BreakpointsForDimension1=|
      | [0; 0.025;
      | 0.051;
      | 0.076;
      | 0.102;
      | 0.127;
      | 0.152;
      | 0.178;
      | 0.203;
      | 0.229;
      | 0.254;
      | 0.279;
      | 0.305
      | ]
      Table=|
      | [0; 124.550;
      | 191.273;
      | 244.652;
      | 284.686;
      | 329.168;
      | 369.202;
      | 391.443;
      | 413.684;
      | 431.477;
      | 449.270;
      | 458.167;
      | 471.511
      | ]
  Rear Rebound min : Lookup_n-D  NumberOfTableDimensions=1  BreakpointsForDimension1=|  Table=|  InternalRulePriority=Speed  RndMeth=Simplest
      BreakpointsForDimension1=|
      | [0; 0.025;
      | 0.051;
      | 0.076;
      | 0.102;
      | 0.127;
      | 0.152;
      | 0.178;
      | 0.203;
      | 0.229;
      | 0.254;
      | 0.279;
      | 0.305
      | ]
      Table=|
      | [0; 35.586;
      | 48.930;
      | 53.379;
      | 53.379;
      | 48.930;
      | 48.930;
      | 48.930;
      | 48.930;
      | 48.930;
      | 48.930;
      | 48.930;
      | 48.930
      | ]
  Saturation : Saturate  UpperLimit=inf  LowerLimit=0
  Saturation1 : Saturate  UpperLimit=0  LowerLimit=-inf
  Subtract : Sum  Inputs=+-
  Subtract1 : Sum  Inputs=+-
  F_RR : Outport
  wires:
  Rear Compression min/1 -> Subtract/2, Add1/2
  Rear Rebound min/1 -> Add2/2, Subtract1/2
  Subtract1/1 -> Gain3/1
  Gain3/1 -> Add2/1
  Subtract/1 -> Gain2/1
  Gain2/1 -> Add1/1
  Rear Compression max/1 -> Subtract/1
  Rear Rebound max/1 -> Subtract1/1
  Saturation/1 -> Rear Compression min/1, Rear Compression max/1
  Gain1/1 -> Rear Rebound min/1, Rear Rebound max/1
  Add2/1 -> Gain/1
  V_RR/1 -> Saturation/1, Saturation1/1
  Saturation1/1 -> Gain1/1
  Gain/1 -> Add/2
  Add1/1 -> Add/1
  Add/1 -> F_RR/1

== system Vehicle_definitivo_validazione_2/Driver in the Loop/Vehicle/Chassis/kinematics/FL ==
  note: mettere 2d su cmaber e toe
  Steer_Angle : Inport
  Wheel_Travel : Inport  Port=2
  Add : Sum
  Add1 : Sum  Inputs=+++
  Anti_dive : Lookup_n-D  NumberOfTableDimensions=1  BreakpointsForDimension1=[-20;-19;-18;-17;-16;-15;-14;-13;-12;-11;-10;-9;-8;-7;-6;-5;-4;-3;-2;-1;0;1;2;3;4;5;6;7;8;9;10;11;12;13;14;15;16;17;18;19;20;21;22;23;24;25;26;27;28;29;30;31;32;33;34;35;36;37;38;39;40;41;42;43;44;45;46;47;48;49;50;51;52;53;54;55;56;57;58;59;60;61;62;63;64;65;66;67;68;69;70;71;72;73;74;75]  Table=[53.85;54.03;54.22;54.4;54.59;54.77;54.96;55.15;55.34;55.53;55.72;55.92;56.11;56.31;56.5;56.7;56.9;57.1;57.3;57.5;57.71;57.91;58.12;58.32;58.53;58.74;58.95;59.16;59.38;59.59;59.81;60.03;60.24;60.46;60.69;60.91;61.13;61.36;61.59;61.81;62.04;62.28;62.51;62.74;62.98;63.22;63.46;63.7;63.94;64.18000000000001;64.43000000000001;64.68000000000001;64.92;65.17;65.43000000000001;65.68000000000001;65.94;66.19;66.45;66.72;66.98;67.23999999999999;67.51000000000001;67.78;68.05;68.31999999999999;68.59999999999999;68.87;69.15000000000001;69.43000000000001;69.72;70;70.29000000000001;70.58;70.87;71.16;71.45999999999999;71.75;72.05;72.36;72.66;72.97;73.28;73.59;73.91;74.22;74.54000000000001;74.86;75.19;75.52;75.84999999999999;76.18000000000001;76.51000000000001;76.84999999999999;77.19;77.54000000000001]/100  InternalRulePriority=Speed  RndMeth=Simplest
  Constant : Constant  Value=car.camber0_front
  Constant1 : Constant  Value=car.toe0_front
  Gain : Gain  Gain=0.222222
  Gain1 : Gain  Gain=-1
  Gain2 : Gain  Gain=-1
  IR : Lookup_n-D  NumberOfTableDimensions=1  BreakpointsForDimension1=[-20;-19;-18;-17;-16;-15;-14;-13;-12;-11;-10;-9;-8;-7;-6;-5;-4;-3;-2;-1;0;1;2;3;4;5;6;7;8;9;10;11;12;13;14;15;16;17;18;19;20;21;22;23;24;25;26;27;28;29;30;31;32;33;34;35;36;37;38;39;40;41;42;43;44;45;46;47;48;49;50;51;52;53;54;55;56;57;58;59;60;61;62;63;64;65;66;67;68;69;70;71;72;73;74;75]  Table=[0.556793;0.557414;0.558036;0.558659;0.559284;0.55991;0.5602240000000001;0.560538;0.561167;0.561167;0.561482;0.561798;0.562114;0.562114;0.562114;0.562114;0.562114;0.562114;0.562114;0.562114;0.561798;0.561798;0.561482;0.561482;0.561167;0.560852;0.560538;0.5602240000000001;0.55991;0.559284;0.558971;0.558347;0.558036;0.557414;0.557103;0.5564829999999999;0.555864;0.555247;0.554631;0.554017;0.553403;0.552792;0.552181;0.551572;0.550661;0.550055;0.549451;0.548546;0.547945;0.547046;0.546448;0.545554;0.544662;0.543774;0.543183;0.542299;0.541419;0.540541;0.539665;0.538793;0.537924;0.537057;0.536193;0.535332;0.534474;0.533618;0.532765;0.531915;0.531067;0.529942;0.529101;0.528262;0.527426;0.526593;0.525486;0.524659;0.523834;0.522739;0.521921;0.521105;0.5202909999999999;0.519211;0.5184029999999999;0.517598;0.516529;0.51573;0.514933;0.514139;0.513084;0.5122949999999999;0.511509;0.510725;0.509944;0.509165;0.508388;0.507614]  InternalRulePriority=Speed  RndMeth=Simplest
  camber : Lookup_n-D  NumberOfTableDimensions=1  BreakpointsForDimension1=[-20;-19;-18;-17;-16;-15;-14;-13;-12;-11;-10;-9;-8;-7;-6;-5;-4;-3;-2;-1;0;1;2;3;4;5;6;7;8;9;10;11;12;13;14;15;16;17;18;19;20;21;22;23;24;25;26;27;28;29;30;31;32;33;34;35;36;37;38;39;40;41;42;43;44;45;46;47;48;49;50;51;52;53;54;55;56;57;58;59;60;61;62;63;64;65;66;67;68;69;70;71;72;73;74;75]  Table=[0.17;0.13;0.08;0.04;-0.01;-0.05;-0.1;-0.15;-0.19;-0.24;-0.29;-0.33;-0.38;-0.42;-0.47;-0.52;-0.5600000000000001;-0.61;-0.66;-0.7;-0.75;-0.8;-0.84;-0.89;-0.9399999999999999;-0.98;-1.03;-1.08;-1.13;-1.17;-1.22;-1.27;-1.31;-1.36;-1.41;-1.46;-1.5;-1.55;-1.6;-1.65;-1.7;-1.74;-1.79;-1.84;-1.89;-1.94;-1.99;-2.03;-2.08;-2.13;-2.18;-2.23;-2.28;-2.33;-2.38;-2.42;-2.47;-2.52;-2.57;-2.62;-2.67;-2.72;-2.77;-2.82;-2.87;-2.92;-2.97;-3.02;-3.07;-3.12;-3.17;-3.23;-3.28;-3.33;-3.38;-3.43;-3.48;-3.53;-3.58;-3.64;-3.69;-3.74;-3.79;-3.84;-3.9;-3.95;-4;-4.05;-4.11;-4.16;-4.21;-4.27;-4.32;-4.37;-4.43;-4.48]+0.75  InternalRulePriority=Speed  RndMeth=Simplest
  steer vs toe ackermann 100% : Lookup_n-D  NumberOfTableDimensions=1  BreakpointsForDimension1=new_lotus_steer.rack_travel  Table=new_lotus_steer.toe_angle_LHS  InternalRulePriority=Speed  RndMeth=Simplest
  steer vs toe1 : Lookup_n-D  NumberOfTableDimensions=1  BreakpointsForDimension1=new_lotus_steer.rack_travel  Table=new_lotus_steer.toe_angle_LHS  InternalRulePriority=Speed  RndMeth=Simplest
  toe : Lookup_n-D  NumberOfTableDimensions=1  BreakpointsForDimension1=[-20;-19;-18;-17;-16;-15;-14;-13;-12;-11;-10;-9;-8;-7;-6;-5;-4;-3;-2;-1;0;1;2;3;4;5;6;7;8;9;10;11;12;13;14;15;16;17;18;19;20;21;22;23;24;25;26;27;28;29;30;31;32;33;34;35;36;37;38;39;40;41;42;43;44;45;46;47;48;49;50;51;52;53;54;55;56;57;58;59;60;61;62;63;64;65;66;67;68;69;70;71;72;73;74;75]  Table=new_lotus_bump.front_LHS.toe  InternalRulePriority=Speed  RndMeth=Simplest
  wheelbase_change : Lookup_n-D  NumberOfTableDimensions=1  BreakpointsForDimension1=[-20;-19;-18;-17;-16;-15;-14;-13;-12;-11;-10;-9;-8;-7;-6;-5;-4;-3;-2;-1;0;1;2;3;4;5;6;7;8;9;10;11;12;13;14;15;16;17;18;19;20;21;22;23;24;25;26;27;28;29;30;31;32;33;34;35;36;37;38;39;40;41;42;43;44;45;46;47;48;49;50;51;52;53;54;55;56;57;58;59;60;61;62;63;64;65;66;67;68;69;70;71;72;73;74;75]  Table=[0.68000000000000005;0.65000000000000002;0.60999999999999999;0.56999999999999995;0.54000000000000004;0.5;0.46999999999999997;0.42999999999999999;0.40000000000000002;0.35999999999999999;0.33000000000000002;0.28999999999999998;0.26000000000000001;0.23000000000000001;0.19;0.16;0.13;0.089999999999999997;0.059999999999999998;0.029999999999999999;0;-0.029999999999999999;-0.059999999999999998;-0.089999999999999997;-0.12;-0.14999999999999999;-0.17999999999999999;-0.20999999999999999;-0.23999999999999999;-0.27000000000000002;-0.29999999999999999;-0.32000000000000001;-0.34999999999999998;-0.38;-0.40000000000000002;-0.42999999999999999;-0.46000000000000002;-0.47999999999999998;-0.51000000000000001;-0.53000000000000003;-0.56000000000000005;-0.57999999999999996;-0.60999999999999999;-0.63;-0.65000000000000002;-0.68000000000000005;-0.69999999999999996;-0.71999999999999997;-0.73999999999999999;-0.76000000000000001;-0.79000000000000004;-0.81000000000000005;-0.82999999999999996;-0.84999999999999998;-0.87;-0.89000000000000001;-0.91000000000000003;-0.92000000000000004;-0.93999999999999995;-0.95999999999999996;-0.97999999999999998;-0.98999999999999999;-1.01;-1.03;-1.04;-1.0600000000000001;-1.0700000000000001;-1.0900000000000001;-1.1000000000000001;-1.1200000000000001;-1.1299999999999999;-1.1399999999999999;-1.1499999999999999;-1.1699999999999999;-1.1799999999999999;-1.1899999999999999;-1.2;-1.21;-1.22;-1.23;-1.24;-1.25;-1.26;-1.26;-1.27;-1.28;-1.29;-1.29;-1.3;-1.3;-1.3100000000000001;-1.3100000000000001;-1.3100000000000001;-1.3200000000000001;-1.3200000000000001;-1.3200000000000001]/1000  InternalRulePriority=Speed  RndMeth=Simplest
  wb_FL : Outport
  AD_FL : Outport  Port=2
  IR_FL : Outport  Port=3
  Camber_FL : Outport  Port=4
  Toe_FL : Outport  Port=5
  wires:
  Wheel_Travel/1 -> Anti_dive/1, IR/1, camber/1, toe/1, wheelbase_change/1
  wheelbase_change/1 -> wb_FL/1
  Anti_dive/1 -> AD_FL/1
  IR/1 -> IR_FL/1
  Constant1/1 -> Add1/1
  Add/1 -> Camber_FL/1
  camber/1 -> Add/2
  Add1/1 -> Toe_FL/1
  Constant/1 -> Add/1
  toe/1 -> Gain2/1
  Steer_Angle/1 -> Gain/1
  Gain/1 -> steer vs toe ackermann 100%/1
  steer vs toe ackermann 100%/1 -> Gain1/1  "toe_FL"
  Gain1/1 -> Add1/3
  Gain2/1 -> Add1/2
